simulink model "InjSys_CtlQnt"  (R2018a)
settings: configuration reference "cs_ert" (kept outside this file)
libraries: simulink x2
settings Model: DataDictionary=InjSys_CtlQnt.sldd  Creator=zhoutinglin  LastModifiedBy=zhoutinglin

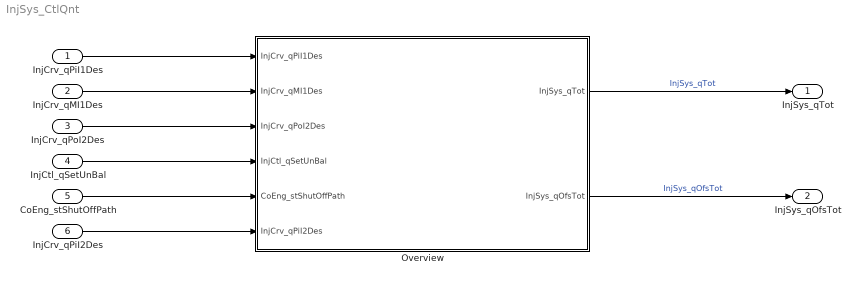
== system InjSys_CtlQnt ==
  InjCrv_qPiI1Des : Inport  Description=Desired PiI injection quantity  OutMin=-319  OutMax=319  OutDataTypeStr=InjMass  Unit=mg/hub  PortDimensions=[1 1]
  InjCrv_qMI1Des : Inport  Description=desired MI1 injection quantity  Port=2  OutMin=-319  OutMax=319  OutDataTypeStr=InjMass  Unit=mg/hub  PortDimensions=[1 1]
  InjCrv_qPoI2Des : Inport  Description=Desired PoI2 injection quantity  Port=3  OutMin=-319  OutMax=319  OutDataTypeStr=InjMass  Unit=mg/hub  PortDimensions=[1 1]
  InjCtl_qSetUnBal : Inport  Description=Current injection quantity  Port=4  OutMin=-319  OutMax=319  OutDataTypeStr=InjMass  Unit=mg/hub  PortDimensions=[1 1]
  CoEng_stShutOffPath : Inport  Description=Active shut-off paths resulting from active reversible,irreversible and afterrun shut-off paths  Port=5  OutMin=0  OutMax=65535  OutDataTypeStr=State2  PortDimensions=[1 1]
  InjCrv_qPiI2Des : Inport  Description=Desired PiI injection quantity  Port=6  OutMin=-319  OutMax=319  OutDataTypeStr=InjMass  Unit=mg/hub  PortDimensions=[1 1]
  Overview : Subsystem
  InjSys_qTot : Outport
  InjSys_qOfsTot : Outport  Port=2
  wires:
  InjCrv_qPiI1Des/1 -> Overview/1(InjCrv_qPiI1Des)
  InjCrv_qMI1Des/1 -> Overview/2(InjCrv_qMI1Des)
  InjCrv_qPoI2Des/1 -> Overview/3(InjCrv_qPoI2Des)
  InjCtl_qSetUnBal/1 -> Overview/4(InjCtl_qSetUnBal)
  CoEng_stShutOffPath/1 -> Overview/5(CoEng_stShutOffPath)
  InjCrv_qPiI2Des/1 -> Overview/6(InjCrv_qPiI2Des)
  Overview/1(InjSys_qTot) -> InjSys_qTot/1  "InjSys_qTot"
  Overview/2(InjSys_qOfsTot) -> InjSys_qOfsTot/1  "InjSys_qOfsTot"

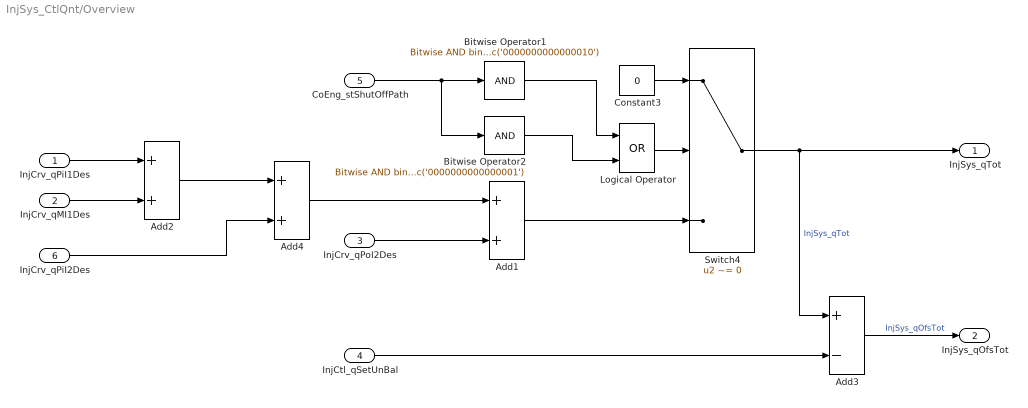
== system InjSys_CtlQnt/Overview ==
  InjCrv_qPiI1Des : Inport  Tag=mg/hub
  InjCrv_qMI1Des : Inport  Tag=mg/hub  Port=2
  InjCrv_qPoI2Des : Inport  Tag=mg/hub  Port=3
  InjCtl_qSetUnBal : Inport  Tag=mg/hub  Port=4
  CoEng_stShutOffPath : Inport  Port=5
  InjCrv_qPiI2Des : Inport  Tag=mg/hub  Port=6
  Add1 : Sum  OutDataTypeStr=Inherit: Inherit via back propagation  SaturateOnIntegerOverflow=on  InputSameDT=on
  Add2 : Sum  OutDataTypeStr=Inherit: Inherit via back propagation  SaturateOnIntegerOverflow=on  InputSameDT=on
  Add3 : Sum  Inputs=+-  OutDataTypeStr=Inherit: Inherit via back propagation  SaturateOnIntegerOverflow=on  InputSameDT=on
  Add4 : Sum  OutDataTypeStr=Inherit: Inherit via back propagation  SaturateOnIntegerOverflow=on  InputSameDT=on
  Bitwise Operator1 : simulink/Logic and Bit Operations/Bitwise Operator  logicop=AND  UseBitMask=on  BitMask=bin2dec('0000000000000010')  BitMaskRealWorld=Stored Integer
  Bitwise Operator2 : simulink/Logic and Bit Operations/Bitwise Operator  logicop=AND  UseBitMask=on  BitMask=bin2dec('0000000000000001')  BitMaskRealWorld=Stored Integer
  Constant3 : Constant  Value=0  OutDataTypeStr=Inherit: Inherit via back propagation
  Logical Operator : Logic  Operator=OR  AllPortsSameDT=off  OutDataTypeStr=boolean
  Switch4 : Switch  Criteria=u2 ~= 0  SaturateOnIntegerOverflow=on  InputSameDT=on
  InjSys_qTot : Outport  Tag=mg/hub
  InjSys_qOfsTot : Outport  Tag=mg/hub  Port=2
  wires:
  InjCtl_qSetUnBal/1 -> Add3/2
  Constant3/1 -> Switch4/1
  InjCrv_qPiI1Des/1 -> Add2/1
  InjCrv_qPoI2Des/1 -> Add1/2
  Bitwise Operator1/1 -> Logical Operator/1
  InjCrv_qMI1Des/1 -> Add2/2
  Add4/1 -> Add1/1
  CoEng_stShutOffPath/1 -> Bitwise Operator1/1, Bitwise Operator2/1
  Add3/1 -> InjSys_qOfsTot/1  "InjSys_qOfsTot"
  Add1/1 -> Switch4/3
  Add2/1 -> Add4/1
  Switch4/1 -> InjSys_qTot/1, Add3/1  "InjSys_qTot"
  Logical Operator/1 -> Switch4/2
  InjCrv_qPiI2Des/1 -> Add4/2
  Bitwise Operator2/1 -> Logical Operator/2
